simulink model "boost_openloop_nss"  (R2026a)
settings: Solver=ode1  StopTime=1.4  FixedStep=5e-06
PreLoadFcn:
  | mdlDir = fileparts(which('boost_openloop_nss'));
  | repoRoot = fileparts(mdlDir);
  | load(fullfile(repoRoot, 'model_data', 'boost_nss_normalized.mat'));
  | load(fullfile(repoRoot, 'model_data', 'comparison_duty_profile.mat'));
  | x0_n = [(6.25 - normStats.y_mean(1)) / normStats.y_std(1); (0.390625 - normStats.y_mean(2)) / normStats.y_std(2)];
libraries: slident x1
settings Model: Creator=arkadiyturevskiy  LastModifiedBy=arkadiyturevskiy

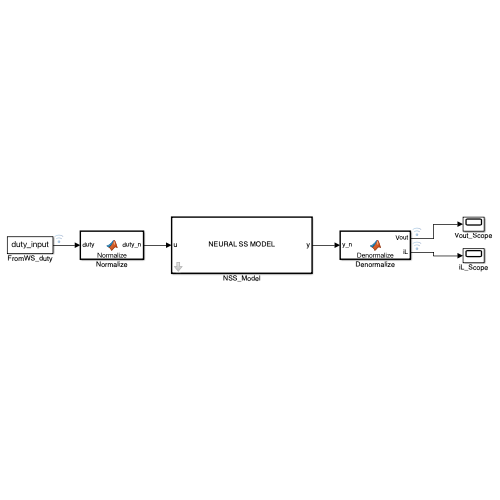
[thumbnail: Simulink's stored preview of the top-level diagram]
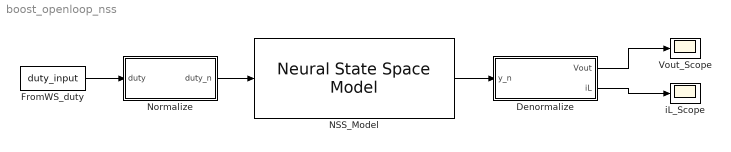
== system boost_openloop_nss ==
  Denormalize : MATLAB Function  TreatAsAtomicUnit=on
  FromWS_duty : FromWorkspace  VariableName=duty_input  OutputAfterFinalValue=Holding final value
  NSS_Model : slident/Models/Neural State Space Model  sys=nssEst  x0type=dialog  ic=x0_n  returnx=off  returndx=off
  Normalize : MATLAB Function  TreatAsAtomicUnit=on
  Vout_Scope : Scope
  iL_Scope : Scope
  wires:
  FromWS_duty/1 -> Normalize/1(duty)
  Normalize/1(duty_n) -> NSS_Model/1
  NSS_Model/1 -> Denormalize/1(y_n)
  Denormalize/1(Vout) -> Vout_Scope/1
  Denormalize/2(iL) -> iL_Scope/1

== matlab function boost_openloop_nss/Normalize ==
  data: duty input; duty_n output
function duty_n = Normalize(duty)
%#codegen
duty_n = (duty - 0.3988994808) / 0.1486619459;

== matlab function boost_openloop_nss/Denormalize ==
  data: y_n input; Vout output; iL output
function [Vout, iL] = Denormalize(y_n)
%#codegen
Vout = y_n(1) * 2.6822801129 + 8.1966344954;
iL   = y_n(2) * 3.3464321089 + 2.9572927340;
